simulink model "FIR_filter0"  (R2020b)
settings: Solver=VariableStepAuto  StartTime=0.0  StopTime=10.0  FixedStep=0.2  RelTol=1e-3
settings Model: Creator=k.Raviteja  LastModifiedBy=k.Raviteja
settings DataIOCC: SaveOutput=off  SaveTime=off

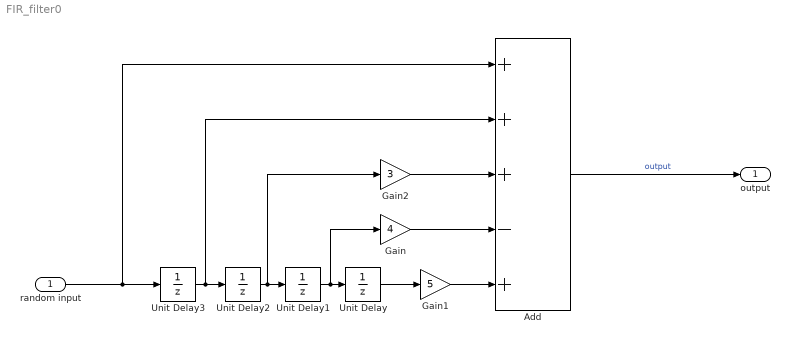
== system FIR_filter0 ==
  random input : Inport  OutDataTypeStr=double  PortDimensions=1  SampleTime=0
  Add : Sum  Inputs=+++-+
  Gain : Gain  Gain=4
  Gain1 : Gain  Gain=5
  Gain2 : Gain  Gain=3
  Unit Delay{,1..3} (4 alike) : UnitDelay  SampleTime=-1  HasFrameUpgradeWarning=on
  output : Outport  OutDataTypeStr=double  PortDimensions=1  SampleTime=0
  wires:
  Unit Delay2/1 -> Gain2/1, Unit Delay1/1
  Gain2/1 -> Add/3
  Add/1 -> output/1  "output"
  Unit Delay/1 -> Gain1/1
  Gain1/1 -> Add/5
  Gain/1 -> Add/4
  Unit Delay3/1 -> Add/2, Unit Delay2/1
  Unit Delay1/1 -> Gain/1, Unit Delay/1
  random input/1 -> Add/1, Unit Delay3/1
